simulink model "iq2xpfb14mcr10"  (R2012b)
settings: Solver=VariableStepDiscrete  SolverMode=SingleTasking  StartTime=0.0  StopTime=10.0  RelTol=1e-3
undefined symbols (not defined in the file or in its folder): pfb_coeff_gen_calc
libraries: xbsIndex_r4 x7581, casper_library_misc x36, casper_library_delays x20, xps_library x6
(part 13 of 90)

== system iq2xpfb14mcr10/fft/fft_biplex/biplex_cplx_unscrambler ==
  even : Inport
  odd : Inport  Port=2
  sync : Inport  Port=3
  Constant : xbsIndex_r4/Constant  const=1  gui_display_data_type=Fixed-point  arith_type=Boolean  n_bits=1  bin_pt=0  preci_type=Single  exp_width=8  frac_width=24  explicit_period=on  period=1  equ=P=C  opselect=C  inp2=PCIN>>17  opr=+  inp1=P  carry=CIN  dbl_ovrd=off  block_type=constant
  Constant1 : xbsIndex_r4/Constant  const=2^(FFTSize-1)  gui_display_data_type=Fixed-point  arith_type=Unsigned  n_bits=FFTSize  bin_pt=0  preci_type=Single  exp_width=8  frac_width=24  explicit_period=on  period=1  equ=P=C  opselect=C  inp2=PCIN>>17  opr=+  inp1=P  carry=CIN  dbl_ovrd=off  block_type=constant
  Constant2 : xbsIndex_r4/Constant  const=2^(FFTSize-1)  gui_display_data_type=Fixed-point  arith_type=Unsigned  n_bits=FFTSize  bin_pt=0  preci_type=Single  exp_width=8  frac_width=24  explicit_period=on  period=1  equ=P=C  opselect=C  inp2=PCIN>>17  opr=+  inp1=P  carry=CIN  dbl_ovrd=off  block_type=constant
  Convert : xbsIndex_r4/Convert  gui_display_data_type=Fixed-point  arith_type=Unsigned  n_bits=1  bin_pt=0  float_type=Single  exp_bits=8  fraction_bits=24  quantization=Truncate  overflow=Wrap  en=off  latency=0  dbl_ovrd=off  pipeline=off  block_type=convert
  Convert1 : xbsIndex_r4/Convert  gui_display_data_type=Fixed-point  arith_type=Unsigned  n_bits=1  bin_pt=0  float_type=Single  exp_bits=8  fraction_bits=24  quantization=Truncate  overflow=Wrap  en=off  latency=0  dbl_ovrd=off  pipeline=off  block_type=convert
  Counter : xbsIndex_r4/Counter  cnt_type=Free Running  cnt_to=Inf  operation=Up  start_count=0  cnt_by_val=1  arith_type=Unsigned  n_bits=FFTSize  bin_pt=0  load_pin=off  rst=on  en=off  explicit_period=off  period=1  dbl_ovrd=off  use_behavioral_HDL=off  implementation=Fabric  use_rpm=on  block_type=counter
  Counter1 : xbsIndex_r4/Counter  cnt_type=Free Running  cnt_to=Inf  operation=Up  start_count=0  cnt_by_val=1  arith_type=Unsigned  n_bits=FFTSize  bin_pt=0  load_pin=off  rst=on  en=off  explicit_period=off  period=1  dbl_ovrd=off  use_behavioral_HDL=off  implementation=Fabric  use_rpm=on  block_type=counter
  Relational : xbsIndex_r4/Relational  mode=a<=b  en=off  latency=0  dbl_ovrd=off  block_type=relational
  Relational1 : xbsIndex_r4/Relational  mode=a<=b  en=off  latency=0  dbl_ovrd=off  block_type=relational
  T0 : Terminator
  T1 : Terminator
  T2 : Terminator
  barrel_switcher : Subsystem  AncestorBlock=casper_library_reorder/barrel_switcher  mask(barrel_switcher){n_inputs=1, async=off}
      mask prompts: n_inputs "Number of Inputs: (2^?)"; async "Asynchronous operation"
      mask help:
      | Shifts input to right by amount specified on sel,
      | wrapping around into higher order bits.
      mask init:
      | barrel_switcher_init(gcb,...
      |     'n_inputs', n_inputs, ...
      |     'async', async);
      mask Help: eval('xlWeb(''http://casper.berkeley.edu/wiki/Barrel_switcher'')')
  barrel_switcher1 : Subsystem  AncestorBlock=casper_library_reorder/barrel_switcher  mask(barrel_switcher){n_inputs=1, async=off}
      mask prompts: n_inputs "Number of Inputs: (2^?)"; async "Asynchronous operation"
      mask help:
      | Shifts input to right by amount specified on sel,
      | wrapping around into higher order bits.
      mask init:
      | barrel_switcher_init(gcb,...
      |     'n_inputs', n_inputs, ...
      |     'async', async);
      mask Help: eval('xlWeb(''http://casper.berkeley.edu/wiki/Barrel_switcher'')')
  reorder : Subsystem  AncestorBlock=casper_library_reorder/reorder  mask(reorder){map=[0 2048 1024 3072 512 2560 1536 3584 256 2304 1280 3328 768 2816 1792 3840 128 2176 1152 3200 640 2688 1664 3712 384 2432 1408 3456 896 2944 1920 3968 64 2112 1088 3136 576 2624 1600 3648 320 2368 1344 3392 832 2880 1856 3904 192 2240 1216 3264 704 2752 1728 3776 448 2496 1472 3520 960 3008 1984 4032 32 2080 1056 3104 544 2592 1568 3616 288 2336 1312 3360 800 2848 1824 3872 160 2208 1184 3232 672 2720 1696 3744 416 2464 1440 3488 928 2976 1952 4000 96 2144 1120 3168 608 2656 1632 3680 352 2400 1376 3424 864 2912 1888 3936 224 2272 1248 3296 736 2784 1760 3808 480 2528 1504 3552 992 3040 2016 4064 16 2064 1040 3088 528 2576 1552 3600 272 2320 1296 3344 784 2832 1808 3856 144 2192 1168 3216 656 2704 1680 3728 400 2448 1424 3472 912 2960 1936 3984 80 2128 1104 3152 592 2640 1616 3664 336 2384 1360 3408 848 2896 1872 3920 208 2256 1232 3280 720 2768 1744 3792 464 2512 1488 3536 976 3024 2000 4048 48 2096 1072 3120 560 2608 1584 3632 304 2352 1328 3376 816 2864 1840 3888 176 2224 1200 3248 688 2736 1712 3760 432 2480 1456 3504 944 2992 1968 4016 112 2160 1136 3184 624 2672 1648 3696 368 2416 1392 3440 880 2928 1904 3952 240 2288 1264 3312 752 2800 1776 3824 496 2544 1520 3568 1008 3056 2032 4080 8 2056 1032 3080 520 2568 1544 3592 264 2312 1288 3336 776 2824 1800 3848 136 2184 1160 3208 648 2696 1672 3720 392 2440 1416 3464 904 2952 1928 3976 72 2120 1096 3144 584 2632 1608 3656 328 2376 1352 3400 840 2888 1864 3912 200 2248 1224 3272 712 2760 1736 3784 456 2504 1480 3528 968 3016 1992 4040 40 2088 1064 3112 552 2600 1576 3624 296 2344 1320 3368 808 2856 1832 3880 168 2216 1192 3240 680 2728 1704 3752 424 2472 1448 3496 936 2984 1960 4008 104 2152 1128 3176 616 2664 1640 3688 360 2408 1384 3432 872 2920 1896 3944 232 2280 1256 3304 744 2792 1768 3816 488 2536 1512 3560 1000 3048 2024 4072 24 2072 1048 3096 536 2584 1560 3608 280 2328 1304 3352 792 2840 1816 3864 152 2200 1176 3224 664 2712 1688 3736 408 2456 1432 3480 920 2968 1944 3992 88 2136 1112 3160 600 2648 1624 3672 344 2392 1368 3416 856 2904 1880 3928 216 2264 1240 3288 728 2776 1752 3800 472 2520 1496 3544 984 3032 2008 4056 56 2104 1080 3128 568 2616 1592 3640 312 2360 1336 3384 824 2872 1848 3896 184 2232 1208 3256 696 2744 1720 3768 440 2488 1464 3512 952 3000 1976 4024 120 2168 1144 3192 632 2680 1656 3704 376 2424 1400 3448 888 2936 1912 3960 248 2296 1272 3320 760 2808 1784 3832 504 2552 1528 3576 1016 3064 2040 4088 4 2052 1028 3076 516 2564 1540 3588 260 2308 1284 3332 772 2820 1796 3844 132 2180 1156 3204 644 2692 1668 3716 388 2436 1412 3460 900 2948 1924 3972 68 2116 1092 3140 580 2628 1604 3652 324 2372 1348 3396 836 2884 1860 3908 196 2244 1220 3268 708 2756 1732 3780 452 2500 1476 3524 964 3012 1988 4036 36 2084 1060 3108 548 2596 1572 3620 292 2340 1316 3364 804 2852 1828 3876 164 2212 1188 3236 676 2724 1700 3748 420 2468 1444 3492 932 2980 1956 4004 100 2148 1124 3172 612 2660 1636 3684 356 2404 1380 3428 868 2916 1892 3940 228 2276 1252 3300 740 2788 1764 3812 484 2532 1508 3556 996 3044 2020 4068 20 2068 1044 3092 532 2580 1556 3604 276 2324 1300 3348 788 2836 1812 3860 148 2196 1172 3220 660 2708 1684 3732 404 2452 1428 3476 916 2964 1940 3988 84 2132 1108 3156 596 2644 1620 3668 340 2388 1364 3412 852 2900 1876 3924 212 2260 1236 3284 724 2772 1748 3796 468 2516 1492 3540 980 3028 2004 4052 52 2100 1076 3124 564 2612 1588 3636 308 2356 1332 3380 820 2868 1844 3892 180 2228 1204 3252 692 2740 1716 3764 436 2484 1460 3508 948 2996 1972 4020 116 2164 1140 3188 628 2676 1652 3700 372 2420 1396 3444 884 2932 1908 3956 244 2292 1268 3316 756 2804 1780 3828 500 2548 1524 3572 1012 3060 2036 4084 12 2060 1036 3084 524 2572 1548 3596 268 2316 1292 3340 780 2828 1804 3852 140 2188 1164 3212 652 2700 1676 3724 396 2444 1420 3468 908 2956 1932 3980 76 2124 1100 3148 588 2636 1612 3660 332 2380 1356 3404 844 2892 1868 3916 204 2252 1228 3276 716 2764 1740 3788 460 2508 1484 3532 972 3020 1996 4044 44 2092 1068 3116 556 2604 1580 3628 300 2348 1324 3372 812 2860 ...(+35853 chars)], n_bits=0, n_inputs=1, bram_latency=bram_latency, map_latency=3, fanout_latency=0, double_buffer=0, bram_map=on}
      mask prompts: map "Output Order:"; n_bits "Data width in"; n_inputs "Number of inputs"; bram_latency "BRAM Latency"; map_latency "Map Latency"; fanout_latency "Fanout latency"; double_buffer "Double Buffer"; bram_map "Use BlockRAM for Map"
      mask init: same as iq2xpfb14mcr10/fft/fft_unscrambler/reorder
      settings: AttributesFormatString=order=2
      mask Help: eval('xlWeb(''http://casper.berkeley.edu/wiki/Reorder'')')
  reorder1 : Subsystem  AncestorBlock=casper_library_reorder/reorder  mask(reorder){map=[4096 6144 5120 7168 4608 6656 5632 7680 4352 6400 5376 7424 4864 6912 5888 7936 4224 6272 5248 7296 4736 6784 5760 7808 4480 6528 5504 7552 4992 7040 6016 8064 4160 6208 5184 7232 4672 6720 5696 7744 4416 6464 5440 7488 4928 6976 5952 8000 4288 6336 5312 7360 4800 6848 5824 7872 4544 6592 5568 7616 5056 7104 6080 8128 4128 6176 5152 7200 4640 6688 5664 7712 4384 6432 5408 7456 4896 6944 5920 7968 4256 6304 5280 7328 4768 6816 5792 7840 4512 6560 5536 7584 5024 7072 6048 8096 4192 6240 5216 7264 4704 6752 5728 7776 4448 6496 5472 7520 4960 7008 5984 8032 4320 6368 5344 7392 4832 6880 5856 7904 4576 6624 5600 7648 5088 7136 6112 8160 4112 6160 5136 7184 4624 6672 5648 7696 4368 6416 5392 7440 4880 6928 5904 7952 4240 6288 5264 7312 4752 6800 5776 7824 4496 6544 5520 7568 5008 7056 6032 8080 4176 6224 5200 7248 4688 6736 5712 7760 4432 6480 5456 7504 4944 6992 5968 8016 4304 6352 5328 7376 4816 6864 5840 7888 4560 6608 5584 7632 5072 7120 6096 8144 4144 6192 5168 7216 4656 6704 5680 7728 4400 6448 5424 7472 4912 6960 5936 7984 4272 6320 5296 7344 4784 6832 5808 7856 4528 6576 5552 7600 5040 7088 6064 8112 4208 6256 5232 7280 4720 6768 5744 7792 4464 6512 5488 7536 4976 7024 6000 8048 4336 6384 5360 7408 4848 6896 5872 7920 4592 6640 5616 7664 5104 7152 6128 8176 4104 6152 5128 7176 4616 6664 5640 7688 4360 6408 5384 7432 4872 6920 5896 7944 4232 6280 5256 7304 4744 6792 5768 7816 4488 6536 5512 7560 5000 7048 6024 8072 4168 6216 5192 7240 4680 6728 5704 7752 4424 6472 5448 7496 4936 6984 5960 8008 4296 6344 5320 7368 4808 6856 5832 7880 4552 6600 5576 7624 5064 7112 6088 8136 4136 6184 5160 7208 4648 6696 5672 7720 4392 6440 5416 7464 4904 6952 5928 7976 4264 6312 5288 7336 4776 6824 5800 7848 4520 6568 5544 7592 5032 7080 6056 8104 4200 6248 5224 7272 4712 6760 5736 7784 4456 6504 5480 7528 4968 7016 5992 8040 4328 6376 5352 7400 4840 6888 5864 7912 4584 6632 5608 7656 5096 7144 6120 8168 4120 6168 5144 7192 4632 6680 5656 7704 4376 6424 5400 7448 4888 6936 5912 7960 4248 6296 5272 7320 4760 6808 5784 7832 4504 6552 5528 7576 5016 7064 6040 8088 4184 6232 5208 7256 4696 6744 5720 7768 4440 6488 5464 7512 4952 7000 5976 8024 4312 6360 5336 7384 4824 6872 5848 7896 4568 6616 5592 7640 5080 7128 6104 8152 4152 6200 5176 7224 4664 6712 5688 7736 4408 6456 5432 7480 4920 6968 5944 7992 4280 6328 5304 7352 4792 6840 5816 7864 4536 6584 5560 7608 5048 7096 6072 8120 4216 6264 5240 7288 4728 6776 5752 7800 4472 6520 5496 7544 4984 7032 6008 8056 4344 6392 5368 7416 4856 6904 5880 7928 4600 6648 5624 7672 5112 7160 6136 8184 4100 6148 5124 7172 4612 6660 5636 7684 4356 6404 5380 7428 4868 6916 5892 7940 4228 6276 5252 7300 4740 6788 5764 7812 4484 6532 5508 7556 4996 7044 6020 8068 4164 6212 5188 7236 4676 6724 5700 7748 4420 6468 5444 7492 4932 6980 5956 8004 4292 6340 5316 7364 4804 6852 5828 7876 4548 6596 5572 7620 5060 7108 6084 8132 4132 6180 5156 7204 4644 6692 5668 7716 4388 6436 5412 7460 4900 6948 5924 7972 4260 6308 5284 7332 4772 6820 5796 7844 4516 6564 5540 7588 5028 7076 6052 8100 4196 6244 5220 7268 4708 6756 5732 7780 4452 6500 5476 7524 4964 7012 5988 8036 4324 6372 5348 7396 4836 6884 5860 7908 4580 6628 5604 7652 5092 7140 6116 8164 4116 6164 5140 7188 4628 6676 5652 7700 4372 6420 5396 7444 4884 6932 5908 7956 4244 6292 5268 7316 4756 6804 5780 7828 4500 6548 5524 7572 5012 7060 6036 8084 4180 6228 5204 7252 4692 6740 5716 7764 4436 6484 5460 7508 4948 6996 5972 8020 4308 6356 5332 7380 4820 6868 5844 7892 4564 6612 5588 7636 5076 7124 6100 8148 4148 6196 5172 7220 4660 6708 5684 7732 4404 6452 5428 7476 4916 6964 5940 7988 4276 6324 5300 7348 4788 6836 5812 7860 4532 6580 5556 7604 5044 7092 6068 8116 4212 6260 5236 7284 4724 6772 5748 7796 4468 6516 5492 7540 4980 7028 6004 8052 4340 6388 5364 7412 4852 6900 5876 7924 4596 6644 5620 7668 5108 7156 6132 8180 4108 6156 5132 7180 4620 6668 5644 7692 4364 6412 5388 7436 4876 6924 5900 7948 4236 6284 5260 7308 4748 6796 5772 7820 4492 6540 5516 7564 5004 7052 6028 ...(+35855 chars)], n_bits=0, n_inputs=1, bram_latency=bram_latency, map_latency=3, fanout_latency=0, double_buffer=0, bram_map=on}
      mask prompts: map "Output Order:"; n_bits "Data width in"; n_inputs "Number of inputs"; bram_latency "BRAM Latency"; map_latency "Map Latency"; fanout_latency "Fanout latency"; double_buffer "Double Buffer"; bram_map "Use BlockRAM for Map"
      mask init: same as iq2xpfb14mcr10/fft/fft_unscrambler/reorder
      settings: AttributesFormatString=order=2
      mask Help: eval('xlWeb(''http://casper.berkeley.edu/wiki/Reorder'')')
  pol1 : Outport
  pol2 : Outport  Port=2
  sync_out : Outport  Port=3
  wires:
  sync/1 -> Counter/1, barrel_switcher/2(sync_in)
  Counter/1 -> Relational/2
  Constant1/1 -> Relational/1
  Relational/1 -> Convert/1
  even/1 -> barrel_switcher/3(In1)
  odd/1 -> barrel_switcher/4(In2)
  Convert/1 -> barrel_switcher/1(sel)
  reorder1/1(sync_out) -> T0/1
  barrel_switcher/1(sync_out) -> reorder/1(sync), reorder1/1(sync)
  barrel_switcher/2(Out1) -> reorder/3(din0)
  barrel_switcher/3(Out2) -> reorder1/3(din0)
  reorder/1(sync_out) -> Counter1/1, barrel_switcher1/2(sync_in)
  reorder/3(dout0) -> barrel_switcher1/3(In1)
  reorder1/3(dout0) -> barrel_switcher1/4(In2)
  Constant2/1 -> Relational1/1
  Counter1/1 -> Relational1/2
  Relational1/1 -> Convert1/1
  Convert1/1 -> barrel_switcher1/1(sel)
  barrel_switcher1/2(Out1) -> pol1/1
  barrel_switcher1/3(Out2) -> pol2/1
  barrel_switcher1/1(sync_out) -> sync_out/1
  reorder1/2(valid) -> T1/1
  reorder/2(valid) -> T2/1
  Constant/1 -> reorder/2(en), reorder1/2(en)
